simulink model "helicecontrolV2"  (R2014b)
settings: Solver=ode14x  StartTime=0.0  StopTime=inf  FixedStep=0.01
undefined symbols (not defined in the file): Serial_Port, Standard_Devices
libraries: rtwinlib x2, dspswit3 x1, fuzblock x1
settings Model: ExtModeTrigDuration=2  Creator=lucasgago  LastModifiedBy=Lucas
settings SolverCC: ZeroCrossControl=DisableAll
settings DebuggingCC: UnderspecifiedInitializationDetection=Classic  MergeDetectMultiDrivingBlocksExec=none  SolverPrmCheckMsg=none
settings HardwareCC: ProdIntDivRoundTo=Zero  ProdEndianess=LittleEndian  ProdHWDeviceType=Generic->32-bit x86 compatible
settings RTWCC: SystemTargetFile=rtwin.tlc  TemplateMakefile=rtwin.tmf  Description=Real-Time Windows Target  RTWVerbose=off  ProcessScript=rtwin_make_rtw_hook  RTWCompilerOptimization=On
settings CodeAppCC: MaxIdLength=95
settings RTWinTargetCC: TargetLibSuffix=_rtwin.lib  TargetPreCompLibLocation=C:\Program Files\MATLAB\R2014b\toolbox\rtw\targets\rtwin\lib\win64

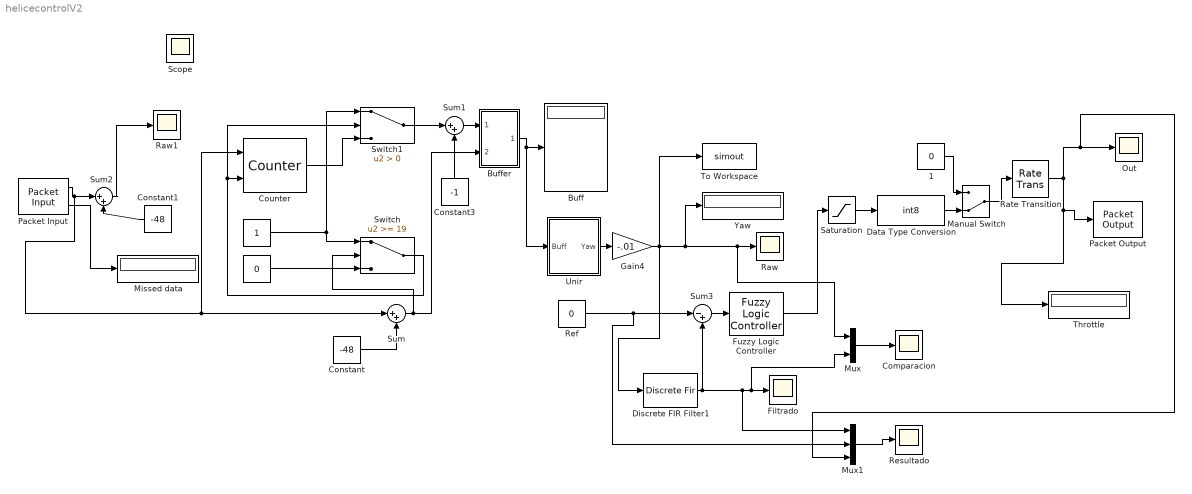
== system helicecontrolV2 ==
  " " : Constant
  "  " : Constant  Value=0
  "  1" : Constant  Value=0
  Buff : Display
  Buffer : Subsystem
  Comparacion : Scope
      settings: TimeRange=3.9  YMin=-25  YMax=25  SaveName=ScopeData6
  Constant : Constant  Value=-48
  Constant1 : Constant  Value=-48
  Constant3 : Constant  Value=-1
  Counter : dspswit3/Counter  Direction=Up  CountEvent=Non-zero sample  CounterSize=User defined  MaxCount=25  InitialCount=0  Output=Count  HitValue=32  ResetInput=on  SamplesPerFrame=1  Ts=1  CntDtype=double  HitDtype=Logical
  Data Type Conversion : DataTypeConversion  OutDataTypeStr=int8
  Discrete FIR Filter1 : DiscreteFir  Coefficients=[0.4 0.3 0.2 0.05 0.03 0.02]
  Filtrado : Scope
      settings: TimeRange=3.9  YMin=-25  YMax=25
  Fuzzy Logic Controller : fuzblock/Fuzzy Logic  Controller  fis=fuzzy_drone
  Gain4 : Gain  Gain=-.01
  Manual Switch : ManualSwitch  CurrentSetting=0
  Missed data : Display
  Mux : Mux  Inputs=2
  Mux1 : Mux  Inputs=3
  Out : Scope
      settings: YMin=59  YMax=66  SaveName=ScopeData4
  Packet Input : rtwinlib/Packet Input  SampleTime=0.01  MaxMissedTicks=100000  ShowMissedTicks=on  YieldWhenWaiting=off  DrvName=Standard_Devices/Serial_Port  DrvAddress=4  DrvOptions=[9600 8 0 0 0 0 0 0]  PacketSize=1  DataTypes='int8'  ShowReady=off  ShowError=off  PacketID=1  ByteOrder=1  ShowTimestamp=off
      settings: AttributesFormatString=Standard Devices\nSerial Port [4h]
  Packet Output : rtwinlib/Packet Output  SampleTime=-1  MaxMissedTicks=10000000  ShowMissedTicks=off  YieldWhenWaiting=off  DrvName=Standard_Devices/Serial_Port  DrvAddress=4  DrvOptions=[9600 8 0 0 0 0 0 0]  PacketSize=1  DataTypes='int8'  ShowReady=off  ShowError=off  PacketID=1  ByteOrder=1  InitialValue=[]  FinalValue=[]
      settings: AttributesFormatString=Standard Devices\nSerial Port [4h]
  Rate Transition : RateTransition
  Raw : Scope
      settings: YMin=-25  YMax=26.5
  Raw1 : Scope
      settings: YMin=0  YMax=20  SaveName=ScopeData2
  Ref : Constant  Value=0
  Resultado : Scope
      settings: TimeRange=3.9  YMin=-25  YMax=25  SaveName=ScopeData7
  Saturation : Saturate  UpperLimit=70  LowerLimit=0
  Sum : Sum  Inputs=|++
  Sum1 : Sum  Inputs=|++
  Sum2 : Sum  Inputs=|++
  Sum3 : Sum  Inputs=|-+
  Switch : Switch  Threshold=19
  Switch1 : Switch  Criteria=u2 > Threshold
  Throttle : Display
  To Workspace : ToWorkspace  VariableName=simout  SampleTime=-1
  Unir : Subsystem
  Yaw : Display
  Scope : Scope
      settings: YMin=-2  YMax=0  SaveName=ScopeData5
  wires:
  Constant/1 -> Sum/2
  Sum/1 -> Switch/2, Buffer/2(Data)
  Counter/1 -> Switch1/3
  "  "/1 -> Switch/3
  " "/1 -> Switch/1, Switch1/1
  Switch/1 -> Switch1/2, Counter/2
  Switch1/1 -> Sum1/1
  Sum1/1 -> Buffer/1(Num)
  Buffer/1(Buff) -> Unir/1(Buff), Buff/1
  Packet Input/1 -> Sum/1, Counter/1, Sum2/1
  Unir/1(Yaw) -> Gain4/1
  Constant3/1 -> Sum1/2
  Gain4/1 -> Yaw/1, Mux/1, Raw/1, To Workspace/1, Discrete FIR Filter1/1
  Discrete FIR Filter1/1 -> Mux1/1, Mux/2, Filtrado/1, Sum3/2
  Constant1/1 -> Sum2/2
  Sum2/1 -> Raw1/1
  Packet Input/2 -> Missed data/1
  Saturation/1 -> Data Type Conversion/1
  Fuzzy Logic Controller/1 -> Saturation/1
  Manual Switch/1 -> Rate Transition/1
  Data Type Conversion/1 -> Manual Switch/2
  "  1"/1 -> Manual Switch/1
  Rate Transition/1 -> Mux1/3, Out/1, Throttle/1, Packet Output/1
  Mux/1 -> Comparacion/1
  Sum3/1 -> Fuzzy Logic Controller/1
  Ref/1 -> Mux1/2, Sum3/1
  Mux1/1 -> Resultado/1

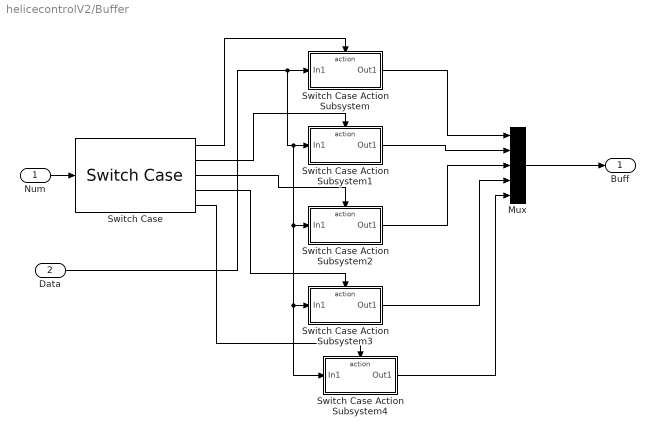
== system helicecontrolV2/Buffer ==
  Num : Inport
  Data : Inport  Port=2
  Mux : Mux  Inputs=5
  Switch Case : SwitchCase  CaseConditions={1,2,3,4,0}  ShowDefaultCase=off
  Switch Case Action Subsystem : Subsystem  TreatAsAtomicUnit=on
  Switch Case Action Subsystem1 : Subsystem  TreatAsAtomicUnit=on
  Switch Case Action Subsystem2 : Subsystem  TreatAsAtomicUnit=on
  Switch Case Action Subsystem3 : Subsystem  TreatAsAtomicUnit=on
  Switch Case Action Subsystem4 : Subsystem  TreatAsAtomicUnit=on
  Buff : Outport
  wires:
  Mux/1 -> Buff/1
  Num/1 -> Switch Case/1
  Switch Case/4 -> Switch Case Action Subsystem3/Action
  Switch Case/3 -> Switch Case Action Subsystem2/Action
  Switch Case/2 -> Switch Case Action Subsystem1/Action
  Switch Case/1 -> Switch Case Action Subsystem/Action
  Switch Case Action Subsystem/1(Out1) -> Mux/1
  Switch Case Action Subsystem1/1(Out1) -> Mux/2
  Switch Case Action Subsystem2/1(Out1) -> Mux/3
  Switch Case Action Subsystem3/1(Out1) -> Mux/4
  Switch Case/5 -> Switch Case Action Subsystem4/Action
  Data/1 -> Switch Case Action Subsystem4/1(In1), Switch Case Action Subsystem3/1(In1), Switch Case Action Subsystem2/1(In1), Switch Case Action Subsystem1/1(In1), Switch Case Action Subsystem/1(In1)
  Switch Case Action Subsystem4/1(Out1) -> Mux/5

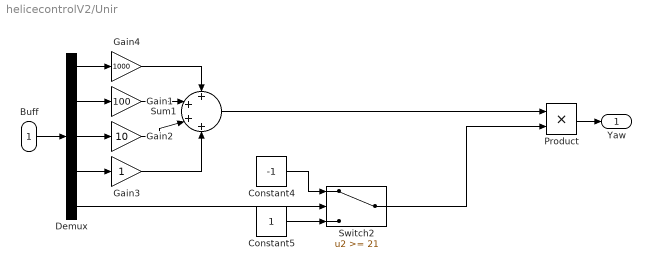
== system helicecontrolV2/Unir ==
  Buff : Inport
  Constant4 : Constant  Value=-1
  Constant5 : Constant
  Demux : Demux  Outputs=5
  Gain1 : Gain  Gain=100
  Gain2 : Gain  Gain=10
  Gain3 : Gain
  Gain4 : Gain  Gain=1000
  Product : Product
  Sum1 : Sum  Inputs=++++
  Switch2 : Switch  Threshold=21
  Yaw : Outport
  wires:
  Gain1/1 -> Sum1/2
  Buff/1 -> Demux/1
  Gain2/1 -> Sum1/3
  Gain3/1 -> Sum1/4
  Gain4/1 -> Sum1/1
  Constant5/1 -> Switch2/3
  Constant4/1 -> Switch2/1
  Product/1 -> Yaw/1
  Demux/1 -> Gain4/1
  Demux/2 -> Gain1/1
  Demux/3 -> Gain2/1
  Demux/4 -> Gain3/1
  Demux/5 -> Switch2/2
  Sum1/1 -> Product/1
  Switch2/1 -> Product/2

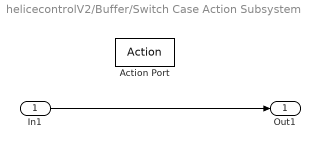
== system helicecontrolV2/Buffer/Switch Case Action Subsystem ==
  In1 : Inport
  Action Port : ActionPort  ActionType=case
  Out1 : Outport
  wires:
  In1/1 -> Out1/1

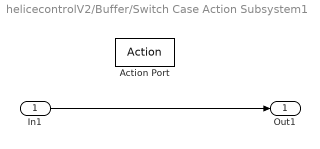
== system helicecontrolV2/Buffer/Switch Case Action Subsystem1 ==
  In1 : Inport
  Action Port : ActionPort  ActionType=case
  Out1 : Outport
  wires:
  In1/1 -> Out1/1

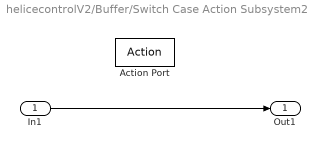
== system helicecontrolV2/Buffer/Switch Case Action Subsystem2 ==
  In1 : Inport
  Action Port : ActionPort  ActionType=case
  Out1 : Outport
  wires:
  In1/1 -> Out1/1

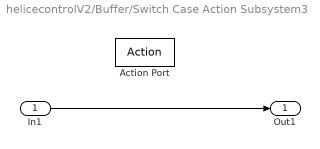
== system helicecontrolV2/Buffer/Switch Case Action Subsystem3 ==
  In1 : Inport
  Action Port : ActionPort  ActionType=case
  Out1 : Outport
  wires:
  In1/1 -> Out1/1

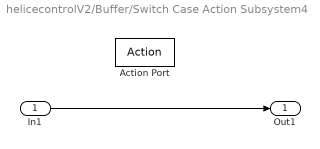
== system helicecontrolV2/Buffer/Switch Case Action Subsystem4 ==
  In1 : Inport
  Action Port : ActionPort  ActionType=case
  Out1 : Outport
  wires:
  In1/1 -> Out1/1
